simulink model "Sim_mono"  (R2023a)
settings: Solver=VariableStepAuto  StartTime=0.0  StopTime=10.0  RelTol=1e-3
values from neighbouring files (symbols this model uses):
  A = double(subs(As))    [Modelo_mono.m]    (also in modelo.mat = [0 0 0 0 0 0 0 0 1 -41.7251957124 0 2.15669687075 ... (64 el; workspace.mat = [0 0 0 0 0 0 0 0 0 0 0 0 ... (64 elements, 8x8)])
  B = double(subs(Bs))    [Modelo_mono.m]    (also in modelo.mat = [0 529.630579069 0 -27.3756082633 0 0 0 0 0 0 0 0 ... (16 el; workspace.mat = [0 0 0 0 50297.8358889 -78.116759971 0 0 0 0 0 0 ... (16 ele)
  K = lqr(Ard,Brd,Qc,Rc)    [Modelo_mono.m]    (also in cascatinha_v3.m = [tprK,0; workspace.mat = [-891.058429104  -1.00065730536e-12  -0.217264538579  -159.5)
  v_ic = [0; 0; 0; 0]    [Modelo_mono.m]    (also in workspace.mat = [0 0 0 0])
  x_ic = [0; 5*pi/180; 0; -5*pi/180]    [Modelo_mono.m]    (also in workspace.mat = [0 0.0872664625997 0 -0.0872664625997])
settings Model: Creator=gabri  LastModifiedBy=pinki
settings OptimizationCC: ReuseModelBlockBuffer=off

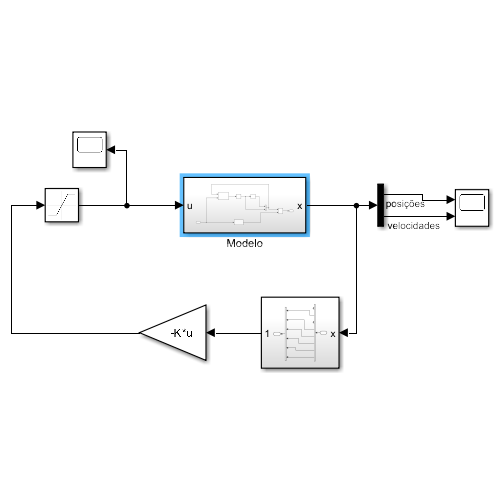
[thumbnail: Simulink's stored preview of the top-level diagram]
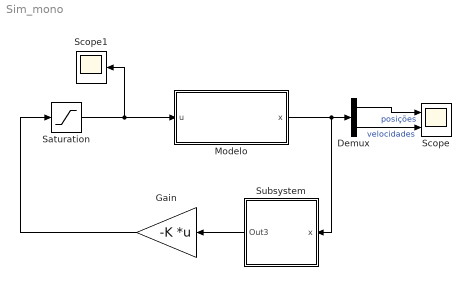
== system Sim_mono ==
  Demux : Demux  Outputs=2
  Gain : Gain  Gain=-K  Multiplication=Matrix(K*u)
  Modelo : Subsystem
  Saturation : Saturate  UpperLimit=1  LowerLimit=-1
  Scope : Scope  NumInputPorts=2
  Scope1 : Scope
  Subsystem : Subsystem
  wires:
  Gain/1 -> Saturation/1
  Subsystem/1(Out3) -> Gain/1
  Modelo/1(x) -> Demux/1, Subsystem/1(x)
  Saturation/1 -> Scope1/1, Modelo/1(u)
  Demux/1 -> Scope/1  "posições"
  Demux/2 -> Scope/2  "velocidades"

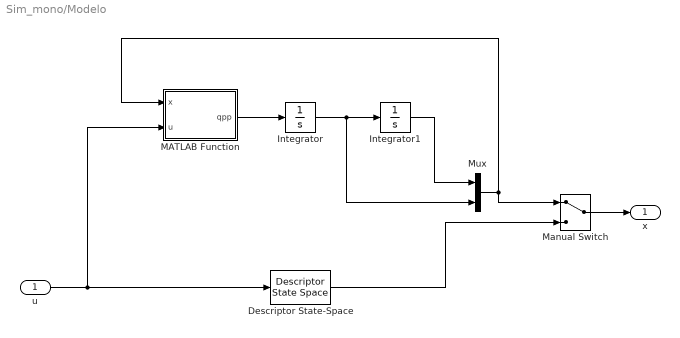
== system Sim_mono/Modelo ==
  u : Inport
  Descriptor State-Space : DescriptorStateSpace  E=eye(8)  A=A  B=B  C=eye(8)  D=zeros(8,2)  InitialCondition=[x_ic; v_ic]
  Integrator : Integrator  InitialCondition=v_ic
  Integrator1 : Integrator  InitialCondition=x_ic
  MATLAB Function : MATLAB Function  TreatAsAtomicUnit=on
  Manual Switch : ManualSwitch
  Mux : Mux  Inputs=2
  x : Outport
  wires:
  Integrator1/1 -> Mux/1
  MATLAB Function/1(qpp) -> Integrator/1
  Integrator/1 -> Mux/2, Integrator1/1
  Mux/1 -> Manual Switch/1, MATLAB Function/1(x)
  u/1 -> MATLAB Function/2(u), Descriptor State-Space/1
  Manual Switch/1 -> x/1
  Descriptor State-Space/1 -> Manual Switch/2

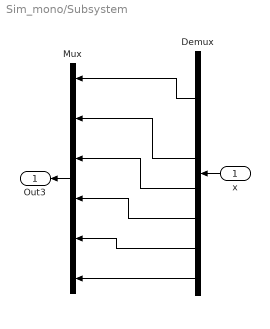
== system Sim_mono/Subsystem ==
  x : Inport
  Demux : Demux  Outputs=8
  Mux : Mux  Inputs=6
  Out3 : Outport
  wires:
  Demux/2 -> Mux/1
  Demux/4 -> Mux/2
  Demux/8 -> Mux/6
  Demux/5 -> Mux/3
  Demux/7 -> Mux/5
  Demux/6 -> Mux/4
  Mux/1 -> Out3/1
  x/1 -> Demux/1

== matlab function Sim_mono/Modelo/MATLAB Function ==
  data: x input; u input; qpp output
function qpp = fcn(x,u)

M = function_M(x(4));
V = function_V(x(6),x(4),x(8),x(5),x(7));
G = function_G(x(2),x(4));
P = function_P();

qpp = M^-1*(-V-G+P*u);
